simulink model "simQuadrotor"  (R2014b)
settings: Solver=ode45  StartTime=0.0  StopTime=tof  FixedStep=dt  MaxStep=dtmax  RelTol=1e-3
values from neighbouring files (symbols this model uses):
  a = (IzzT - IxxT)./ IxxT    [quadrotor.m]
  alpha = 1    [quadrotor.m]
  Aq = -20    [quadrotor.m]
  Ar = -10*eye(2)    [quadrotor.m]
  Arm = [-20 0 ; 0 -5]    [quadrotor.m]
  As = -50*eye(3)    [quadrotor.m]
  attitudeControlFlag = 4    [quadrotor.m]
  Bq = 1    [quadrotor.m]
  Br = [1 0]    [quadrotor.m]
  Dhat0 = zeros(3,1)    [quadrotor.m]
  Dlimit = 2.5    [quadrotor.m]
  DSecondLimit = 2    [quadrotor.m]
  dtFc = 10e-3    (= 0.01)    [quadrotor.m]
  epsilon = 0.1    [quadrotor.m]
  epsilontheta = 0.1    [quadrotor.m]
  euler0 = [0 0 0]'*pi/180    [quadrotor.m]
  Eulerc_ftc = [0 0 0]'    [quadrotor.m]
  faultyPropellerVec = double(not(faultyPropellerVec))    [quadrotor.m]
  FDstart = 3    [quadrotor.m]
  flims = [0.2*0 3.8*2.5]    [quadrotor.m]
  ftc_f2 = 0.1*2    (= 0.2)    [quadrotor.m]
  g = 9.81    [quadrotor.m]
  GammaW = 10000    [quadrotor.m]
  IxxB = IxxT - 4*IxxP    (= 0.0027)    [quadrotor.m]
  IxxT = 2.7e-3    (= 0.0027)    [quadrotor.m]
  IyyB = IyyT - 4*IyyP    (= 0.0027)    [quadrotor.m]
  IyyT = IxxT    (= 0.0027)    [quadrotor.m]
  IzzB = IzzT - 4*IzzP    (= 0.00514)    [quadrotor.m]
  IzzP = 1.5e-5    (= 1.5e-05)    [quadrotor.m]
  IzzT = 5.2e-3    (= 0.0052)    [quadrotor.m]
  Kdxx = 0.7e-4/10    (= 7e-06)    [quadrotor.m]
  Kdzz = 1.4e-4    (= 0.00014)    [quadrotor.m]
  Kf = 6.41e-6    (= 6.41e-06)    [quadrotor.m]
  Kp = 2*0.75*diag([1 1 1])    [quadrotor.m]
  Kp4 = 0.05    [quadrotor.m]
  Ktau = 1.72e-2    (= 0.0172)    [quadrotor.m]
  Kv = 0*0.005*diag([1 1 1])    [quadrotor.m]
  Kv4 = 0.02    [quadrotor.m]
  l = 0.17    [quadrotor.m]
  m = 0.5    [quadrotor.m]
  nc_ftc = 1    [quadrotor.m]
  nCheby = 3    [quadrotor.m]
  pqr0 = [0 0 0]'*pi/180    [quadrotor.m]
  Ps = lyap(As',Q)    [quadrotor.m]
  q0 = [euler0 ; pqr0]    [quadrotor.m]
  qp0 = 0    [quadrotor.m]
  sigmaMot = 0.015    [quadrotor.m]
  tfault = 5    [quadrotor.m]
  Vb0 = [0 0 0]'    [quadrotor.m]
  W0 = 0    [quadrotor.m]
  Wbnd = 10    [quadrotor.m]
  Xe0 = [0 0 0]'    [quadrotor.m]
  xhat0 = [pqr0]    [quadrotor.m]
undefined symbols (not defined in the file or in its folder): Intmax, Intmin, magnitude, rmax, rmin
libraries: aerolibutil x38, simulink x11, vrlib x3, dspbuff3 x1
(part 1 of 3)
settings Model: Creator=alp.marangoz  LastModifiedBy=alpmarangoz
settings SolverCC: AutoInsertRateTranBlk=on
settings DataIOCC: SignalLoggingSaveFormat=ModelDataLogs
settings OptimizationCC: ExpressionDepthLimit=2147483647
settings DebuggingCC: UnderspecifiedInitializationDetection=Classic  MergeDetectMultiDrivingBlocksExec=none  InheritedTsInSrcMsg=none  CheckMatrixSingularityMsg=error  FcnCallInpInsideContextMsg=UseLocalSettings  StateNameClashWarn=warning
settings GRTTargetCC: CombineOutputUpdateFcns=off  GRTInterface=on

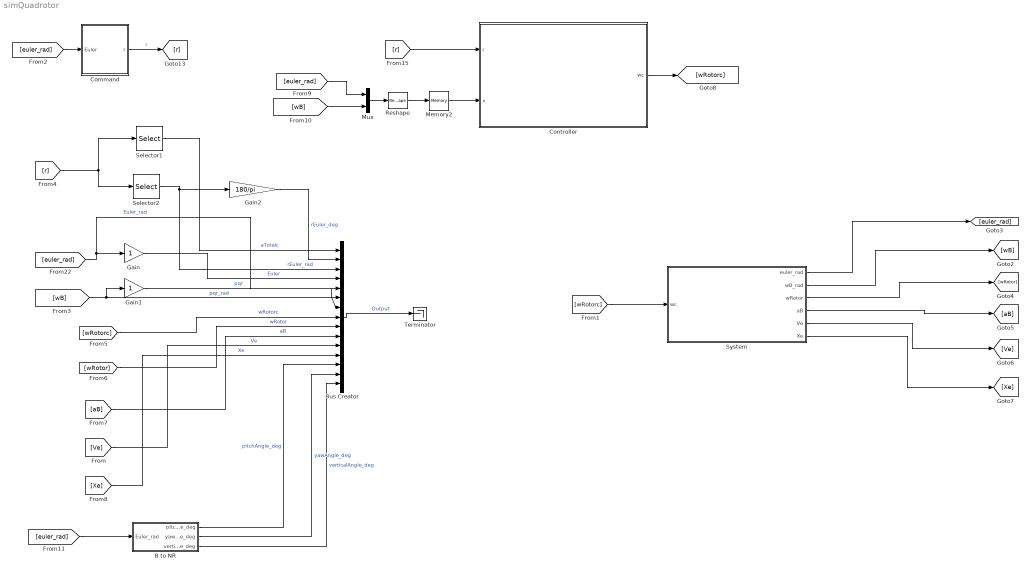
== system simQuadrotor ==
  B to NR : Subsystem  TreatAsAtomicUnit=on
  Bus Creator : BusCreator  Inputs=15
  Command : Subsystem  TreatAsAtomicUnit=on  SystemSampleTime=dtFc
  Controller : Subsystem  TreatAsAtomicUnit=on  SystemSampleTime=dtFc
  Gain : Gain
  Gain1 : Gain
  Gain2 : Gain  Gain=180/pi
  Memory2 : Memory  X0=q0  InheritSampleTime=on  LinearizeMemory=on  LinearizeAsDelay=on
  Mux : Mux  Inputs=2
  Reshape : Reshape  OutputDimensionality=Column vector (2-D)
  Selector1 : Selector  NumberOfDimensions=2  InputPortWidth=2  IndexOptions=Index vector (dialog),Index vector (dialog)  Indices=1,1  OutputSizes=1,1
  Selector2 : Selector  NumberOfDimensions=2  InputPortWidth=3  IndexOptions=Index vector (dialog),Index vector (dialog)  Indices=[2 3 4],1  OutputSizes=1,1
  System : Subsystem  TreatAsAtomicUnit=on
  Terminator : Terminator
  wires:
  Command/1(r) -> [r]  "r"
  Controller/1(wc) -> [wRotorc]
  [wRotorc] -> System/1(wc)
  Reshape/1 -> Memory2/1
  [euler_rad] -> Command/1(Euler)
  Memory2/1 -> Controller/2(x)
  [r] -> Controller/1(r)
  Bus Creator/1 -> Terminator/1  "Output"
  [r] -> Selector1/1, Selector2/1
  System/3(wRotor) -> [wRotor]
  System/4(aB) -> [aB]
  System/5(Ve) -> [Ve]
  System/6(Xe) -> [Xe]
  Selector1/1 -> Bus Creator/1  "aTotalc"
  Selector2/1 -> Gain2/1, Bus Creator/3  "rEuler_rad"
  [euler_rad] -> Gain/1, Bus Creator/5  "Euler_rad"
  [wRotorc] -> Bus Creator/8  "wRotorc"
  [wRotor] -> Bus Creator/9  "wRotor"
  [aB] -> Bus Creator/10  "aB"
  [Ve] -> Bus Creator/11  "Ve"
  [Xe] -> Bus Creator/12  "Xe"
  System/1(euler_rad) -> [euler_rad]
  System/2(wB_rad) -> [wB]
  Mux/1 -> Reshape/1
  [euler_rad] -> Mux/1
  [wB] -> Mux/2
  Gain/1 -> Bus Creator/4  "Euler"
  [wB] -> Bus Creator/7, Gain1/1  "pqr_rad"
  Gain1/1 -> Bus Creator/6  "pqr"
  [euler_rad] -> B to NR/1(Euler_rad)
  B to NR/1(pitchAngle_deg) -> Bus Creator/13  "pitchAngle_deg"
  B to NR/2(yawAngle_deg) -> Bus Creator/14  "yawAngle_deg"
  B to NR/3(verticalAngle_deg) -> Bus Creator/15  "verticalAngle_deg"
  Gain2/1 -> Bus Creator/2  "rEuler_deg"

== system simQuadrotor/B to NR ==
  Euler_rad : Inport
  Add : Sum
  Add1 : Sum  Inputs=+-
  Constant1 : Constant  Value=90  VectorParams1D=off
  Constant2 : Constant  Value=[0 0 1]'  VectorParams1D=off
  DCM E to B1 : Subsystem
  Gain : Gain  Gain=180/pi
  Gain1 : Gain  Gain=180/pi
  Math Function : Math  Operator=square  SaturateOnIntegerOverflow=on
  Math Function1 : Math  Operator=square  SaturateOnIntegerOverflow=on
  Math Function2 : Math  Operator=transpose  SaturateOnIntegerOverflow=on
  Product4 : Product  Multiplication=Matrix(*)  RndMeth=Zero
  Selector1 : Selector  InputPortWidth=3  Indices=3
  Selector2 : Selector  InputPortWidth=3  Indices=2
  Selector3 : Selector  InputPortWidth=3
  Sqrt : Sqrt  SaturateOnIntegerOverflow=on
  Trigonometric Function : Trigonometry  Operator=atan2
  Trigonometric Function1 : Trigonometry  Operator=atan2
  pitchAngle_deg : Outport
  yawAngle_deg : Outport  Port=2
  verticalAngle_deg : Outport  Port=3
  wires:
  Euler_rad/1 -> [phithetapsi]  "Euler_rad"
  Math Function2/1 -> [R]
  [phithetapsi] -> DCM E to B1/1(phithetapsi)
  DCM E to B1/1(CB_E) -> Math Function2/1
  [R] -> Product4/1
  Constant2/1 -> Product4/2
  Product4/1 -> [Gamma]
  [Gamma] -> Selector1/1, Selector3/1, Selector2/1
  Selector3/1 -> [u1]
  Selector2/1 -> [u2]
  Selector1/1 -> [u3]
  [u1] -> Math Function/1
  [u2] -> Math Function1/1
  Math Function/1 -> Add/1
  Math Function1/1 -> Add/2
  Add/1 -> Sqrt/1
  [u3] -> Trigonometric Function/1
  Sqrt/1 -> Trigonometric Function/2
  Trigonometric Function/1 -> Gain/1
  Trigonometric Function1/1 -> Gain1/1
  [u2] -> Trigonometric Function1/1
  [u1] -> Trigonometric Function1/2
  [yawAngle_deg] -> yawAngle_deg/1
  [pitchAngle_deg] -> pitchAngle_deg/1
  Gain/1 -> [pitchAngle_deg]
  Gain1/1 -> [yawAngle_deg]
  Constant1/1 -> Add1/2
  [pitchAngle_deg] -> Add1/1
  Add1/1 -> [verticalAngle_deg]
  [verticalAngle_deg] -> verticalAngle_deg/1

== system simQuadrotor/Command ==
  Euler : Inport
  From Workspace : FromWorkspace  VariableName=r  Interpolate=off  OutputAfterFinalValue=Setting to zero
  Memory2 : Memory  X0=euler0  InheritSampleTime=on  LinearizeMemory=on  LinearizeAsDelay=on
  Reshape1 : Reshape  OutputDimensionality=Column vector (2-D)
  Selector : Selector  NumberOfDimensions=2  InputPortWidth=2  IndexOptions=Index vector (dialog),Index vector (dialog)  Indices=1,1  OutputSizes=1,1
  Selector1 : Selector  NumberOfDimensions=2  InputPortWidth=3  IndexOptions=Index vector (dialog),Index vector (dialog)  Indices=[2 3 4],1  OutputSizes=1,1
  Subtract : Sum  Inputs=+-
  Terminator : Terminator
  Terminator1 : Terminator
  Terminator2 : Terminator
  r : Outport  InitialOutput=0
  wires:
  From Workspace/1 -> Reshape1/1
  Reshape1/1 -> r/1, Selector/1, Selector1/1
  Euler/1 -> Memory2/1
  Memory2/1 -> [euler]
  [euler] -> Subtract/2  "q"
  Selector/1 -> Terminator/1  "rnc"
  Selector1/1 -> Terminator2/1, Subtract/1  "rEuler"
  Subtract/1 -> Terminator1/1  "eEuler"

== system simQuadrotor/Controller ==
  r : Inport
  x : Inport  Port=2
  1 : Selector  NumberOfDimensions=2  InputPortWidth=4  IndexOptions=Index vector (dialog),Index vector (dialog)  Indices=[1],1  OutputSizes=1,1
  2 : Selector  NumberOfDimensions=2  InputPortWidth=4  IndexOptions=Index vector (dialog),Index vector (dialog)  Indices=[2 3 4],1  OutputSizes=1,1
  Disturbance Estimator : Subsystem
  FTC Controller : Subsystem  TreatAsAtomicUnit=on
  Fault Detection : Subsystem  TreatAsAtomicUnit=on
  Gain : Gain  Gain=180/pi
  Gain1 : Gain
  Logical Operator : Logic  Operator=NOT  AllPortsSameDT=off  OutDataTypeStr=boolean
  Memory1 : Memory  InheritSampleTime=on  LinearizeMemory=on  LinearizeAsDelay=on
  Memory2 : Memory  InheritSampleTime=on  LinearizeMemory=on  LinearizeAsDelay=on
  Memory3 : Memory  InheritSampleTime=on  LinearizeMemory=on  LinearizeAsDelay=on
  Nominal Controller : Subsystem  TreatAsAtomicUnit=on
  Reshape3 : Reshape  OutputDimensionality=Column vector (2-D)
  Switch : Switch  Criteria=u2 > Threshold
  Terminator : Terminator
  Terminator1 : Terminator
  Terminator2 : Terminator
  "[4 5 6]" : Selector  NumberOfDimensions=2  InputPortWidth=3  IndexOptions=Index vector (dialog),Index vector (dialog)  Indices=[4 5 6],1  OutputSizes=1,1
  wc : Outport
  wires:
  r/1 -> [r]  "r"
  x/1 -> [x]  "x"
  [wc] -> wc/1  "wc"
  [x] -> "[4 5 6]"/1
  "[4 5 6]"/1 -> Reshape3/1
  Reshape3/1 -> Terminator2/1  "pqr"
  Switch/1 -> [wc]
  [wcNominal] -> Switch/3
  [wcFTC] -> Gain1/1
  [faultDetected] -> Switch/2  "faultDetected"
  [r] -> 1/1, 2/1
  1/1 -> Terminator1/1  "nc"
  2/1 -> Gain/1
  Gain/1 -> Terminator/1  "Eulerc"
  [r] -> Nominal Controller/1(r)
  [x] -> Nominal Controller/2(x)
  Nominal Controller/1(wcNominal) -> [wcNominal]  "wcNominal"
  Logical Operator/1 -> Memory2/1
  Memory1/1 -> [enableFTC]
  Memory2/1 -> [enableNominal]
  [faultDetected] -> Logical Operator/1, Memory1/1
  [enableNominal] -> Nominal Controller/Enable
  [enableFTC] -> FTC Controller/Enable
  [x] -> FTC Controller/2(x)
  FTC Controller/1(wcFTC) -> [wcFTC]  "wcFTC"
  Gain1/1 -> Switch/1
  Disturbance Estimator/1(Dhat) -> [Dhat]
  [Dhat] -> Fault Detection/1(Dhat)
  Fault Detection/2(faultDetected) -> [faultDetected]
  [enableNominal] -> Disturbance Estimator/Enable
  Fault Detection/1(faultyRotor) -> [faultyRotor]
  [faultyRotor] -> FTC Controller/1(faultyRotor)
  [wc] -> Memory3/1
  Memory3/1 -> Disturbance Estimator/2(wc)
  [x] -> Disturbance Estimator/1(x)

== system simQuadrotor/System ==
  wc : Inport
  Demux : Demux
  Fault Insertion : Subsystem
  Flight Mechanics : Subsystem
  Gain7 : Gain  Gain=Kf
  Math Function7 : Math  Operator=magnitude^2  SaturateOnIntegerOverflow=on
  Motor Dynamics : Subsystem
  Navigation : Subsystem
  Reshape5 : Reshape  OutputDimensionality=Column vector (2-D)
  Terminator : Terminator
  euler_rad : Outport
  wB_rad : Outport  Port=2
  wRotor : Outport  Port=3
  aB : Outport  Port=4
  Ve : Outport  Port=5
  Xe : Outport  Port=6
  wires:
  wc/1 -> Reshape5/1
  Reshape5/1 -> [wc]  "wc"
  [euler_rad] -> euler_rad/1
  Flight Mechanics/1(aB) -> [aB], Navigation/1(axyz)
  Flight Mechanics/2(wB_rad) -> Navigation/2(wxyz), [wB]
  [wc] -> Demux/1
  Demux/1 -> Motor Dynamics/1(w1c)
  Demux/2 -> Motor Dynamics/2(w2c)
  Demux/3 -> Motor Dynamics/3(w3c)
  Demux/4 -> Motor Dynamics/4(w4c)
  [euler_rad] -> Flight Mechanics/5(Euler)
  Navigation/1(Ve) -> [Ve]
  Navigation/2(Xe) -> [Xe]
  Navigation/3(euler_rad) -> [euler_rad]
  [wRotor] -> wRotor/1
  [Xe] -> Xe/1
  [Ve] -> Ve/1
  [aB] -> aB/1
  Motor Dynamics/1(wRotor) -> Fault Insertion/1(wRotor)
  Fault Insertion/1(wRotor_app) -> Math Function7/1, [wRotor]
  Fault Insertion/5(w4) -> Flight Mechanics/4(w4)
  Fault Insertion/4(w3) -> Flight Mechanics/3(w3)
  Fault Insertion/3(w2) -> Flight Mechanics/2(w2)
  Fault Insertion/2(w1) -> Flight Mechanics/1(w1)
  [wB] -> wB_rad/1
  Gain7/1 -> Terminator/1  "frotorApp"
  Math Function7/1 -> Gain7/1

== system simQuadrotor/B to NR/DCM E to B1 ==
  phithetapsi : Inport
  Create 3x3 Matrix : aerolibutil/Create 3x3 Matrix
  Fcn11 : Fcn  Expr=u(5)*u(6)
  Fcn12 : Fcn  Expr=u(3)*u(5)
  Fcn13 : Fcn  Expr=-u(2)
  Fcn21 : Fcn  Expr=u(1)*u(2)*u(6)-u(4)*u(3)
  Fcn22 : Fcn  Expr=u(1)*u(2)*u(3)+u(4)*u(6)
  Fcn23 : Fcn  Expr=u(1)*u(5)
  Fcn31 : Fcn  Expr=u(4)*u(2)*u(6)+u(1)*u(3)
  Fcn32 : Fcn  Expr=u(4)*u(2)*u(3)-u(1)*u(6)
  Fcn33 : Fcn  Expr=u(4)*u(5)
  Mux : Mux  Inputs=2
  sincos : Trigonometry  Operator=sincos
  CB_E : Outport
  wires:
  Create 3x3 Matrix/1 -> CB_E/1  "CB_E"
  phithetapsi/1 -> sincos/1  "phithetapsi"
  Fcn33/1 -> Create 3x3 Matrix/9
  Fcn32/1 -> Create 3x3 Matrix/8
  Fcn23/1 -> Create 3x3 Matrix/6
  Fcn22/1 -> Create 3x3 Matrix/5
  Fcn31/1 -> Create 3x3 Matrix/7
  Fcn21/1 -> Create 3x3 Matrix/4
  Fcn13/1 -> Create 3x3 Matrix/3
  Fcn12/1 -> Create 3x3 Matrix/2
  Fcn11/1 -> Create 3x3 Matrix/1
  Mux/1 -> Fcn21/1, Fcn13/1, Fcn12/1, Fcn11/1, Fcn22/1, Fcn23/1, Fcn31/1, Fcn33/1, Fcn32/1
  sincos/2 -> Mux/2
  sincos/1 -> Mux/1

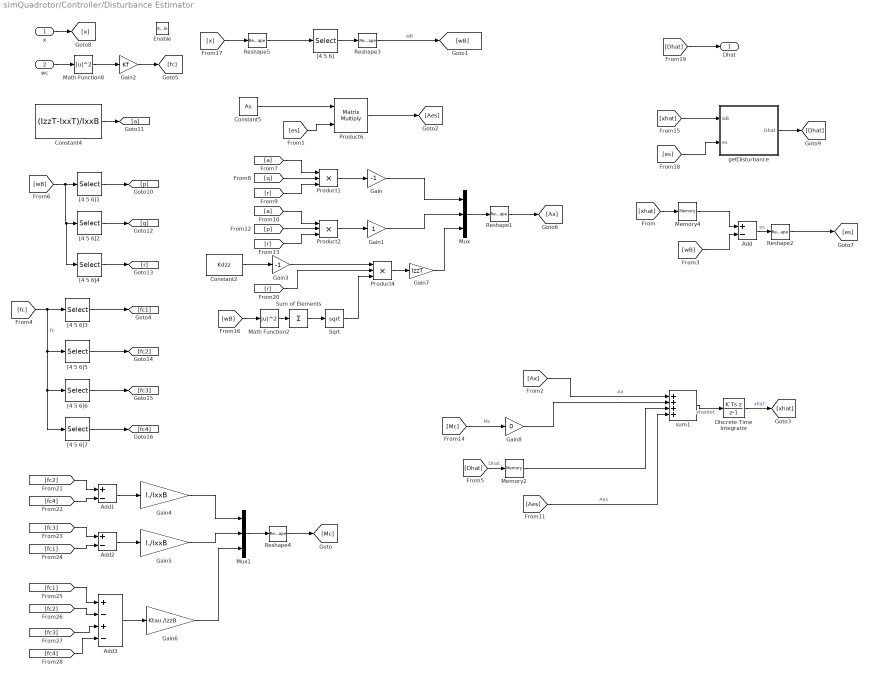
== system simQuadrotor/Controller/Disturbance Estimator ==
  x : Inport
  wc : Inport  Port=2
  Enable : EnablePort
  Add : Sum  Inputs=+-
  Add1 : Sum  Inputs=+-
  Add2 : Sum  Inputs=+-
  Add3 : Sum  Inputs=+-+-
  Constant2 : Constant  Value=Kdzz  VectorParams1D=off
  Constant4 : Constant  Value=(IzzT-IxxT)/IxxB  VectorParams1D=off
  Constant5 : Constant  Value=As
  Discrete-Time Integrator : DiscreteIntegrator  IntegratorMethod=Integration: Backward Euler  InitialCondition=xhat0  InitialConditionSetting=State (most efficient)  SampleTime=-1  UpperSaturationLimit=Intmax  LowerSaturationLimit=Intmin
  Gain : Gain  Gain=-1
  Gain1 : Gain
  Gain2 : Gain  Gain=Kf
  Gain3 : Gain  Gain=-1
  Gain4 : Gain  Gain=l./IxxB
  Gain5 : Gain  Gain=l./IxxB
  Gain6 : Gain  Gain=Ktau./IzzB
  Gain7 : Gain  Gain=IzzT
  Gain8 : Gain  Gain=0
  Math Function2 : Math  Operator=magnitude^2  SaturateOnIntegerOverflow=on
  Math Function8 : Math  Operator=magnitude^2  SaturateOnIntegerOverflow=on
  Memory2 : Memory  X0=Dhat0  InheritSampleTime=on  LinearizeMemory=on  LinearizeAsDelay=on
  Memory4 : Memory  X0=xhat0  InheritSampleTime=on  LinearizeMemory=on  LinearizeAsDelay=on
  Mux : Mux  Inputs=3
  Mux1 : Mux  Inputs=3
  Product1 : Product  Inputs=3  RndMeth=Zero
  Product2 : Product  Inputs=3  RndMeth=Zero
  Product4 : Product  Inputs=3  RndMeth=Zero
  Product6 : Product  Multiplication=Matrix(*)  RndMeth=Zero
  Reshape{1..5} (5 alike) : Reshape  OutputDimensionality=Column vector (2-D)
  Sqrt : Sqrt  SaturateOnIntegerOverflow=on
  Sum of Elements : Sum  Inputs=+
  "[4 5 6]" : Selector  NumberOfDimensions=2  InputPortWidth=3  IndexOptions=Index vector (dialog),Index vector (dialog)  Indices=[4 5 6],1  OutputSizes=1,1
  "[4 5 6]1" : Selector  InputPortWidth=3
  "[4 5 6]2" : Selector  InputPortWidth=3  Indices=2
  "[4 5 6]3" : Selector  InputPortWidth=4
  "[4 5 6]4" : Selector  InputPortWidth=3  Indices=3
  "[4 5 6]5" : Selector  InputPortWidth=4  Indices=2
  "[4 5 6]6" : Selector  InputPortWidth=4  Indices=3
  "[4 5 6]7" : Selector  InputPortWidth=4  Indices=4
  getDisturbance : Subsystem
  sum1 : Sum  Inputs=++++
  Dhat : Outport
  wires:
  [xhat] -> getDisturbance/1(wB)
  [es] -> getDisturbance/2(es)
  getDisturbance/1(Dhat) -> [Dhat]
  [Dhat] -> Dhat/1
  Constant4/1 -> [a]
  x/1 -> [x]
  [x] -> Reshape5/1
  "[4 5 6]"/1 -> Reshape3/1
  Reshape5/1 -> "[4 5 6]"/1
  Reshape3/1 -> [wB]  "wB"
  Product6/1 -> [Aes]
  Constant5/1 -> Product6/1
  [es] -> Product6/2
  Reshape2/1 -> [es]
  [xhat] -> Memory4/1
  [wB] -> Add/2
  Add/1 -> Reshape2/1  "es"
  Memory4/1 -> Add/1
  [Dhat] -> Memory2/1  "Dhat"
  [Ax] -> sum1/1  "Ax"
  sum1/1 -> Discrete-Time Integrator/1  "xhatdot"
  Discrete-Time Integrator/1 -> [xhat]  "xhat"
  [wB] -> "[4 5 6]4"/1, "[4 5 6]2"/1, "[4 5 6]1"/1
  "[4 5 6]2"/1 -> [q]
  "[4 5 6]1"/1 -> [p]
  "[4 5 6]4"/1 -> [r]
  Reshape1/1 -> [Ax]
  Mux/1 -> Reshape1/1
  [q] -> Product1/2
  [r] -> Product1/3
  [a] -> Product1/1
  [p] -> Product2/2
  [r] -> Product2/3
  [a] -> Product2/1
  Product1/1 -> Gain/1
  Gain/1 -> Mux/1
  Product2/1 -> Gain1/1
  Gain1/1 -> Mux/2
  Product4/1 -> Gain7/1
  [Mc] -> Gain8/1  "Mc"
  wc/1 -> Math Function8/1
  Math Function8/1 -> Gain2/1
  Gain2/1 -> [fc]
  Memory2/1 -> sum1/3
  [Aes] -> sum1/4  "Aes"
  [r] -> Product4/2
  Gain3/1 -> Product4/1
  Constant2/1 -> Gain3/1
  Math Function2/1 -> Sum of Elements/1
  Sum of Elements/1 -> Sqrt/1
  [wB] -> Math Function2/1
  Sqrt/1 -> Product4/3
  Reshape4/1 -> [Mc]
  Mux1/1 -> Reshape4/1
  [fc] -> "[4 5 6]7"/1, "[4 5 6]6"/1, "[4 5 6]5"/1, "[4 5 6]3"/1  "fc"
  "[4 5 6]3"/1 -> [fc1]
  "[4 5 6]5"/1 -> [fc2]
  "[4 5 6]6"/1 -> [fc3]
  "[4 5 6]7"/1 -> [fc4]
  [fc2] -> Add1/1
  [fc4] -> Add1/2
  Add1/1 -> Gain4/1
  Gain4/1 -> Mux1/1
  [fc3] -> Add2/1
  [fc1] -> Add2/2
  Add2/1 -> Gain5/1
  Gain5/1 -> Mux1/2
  [fc1] -> Add3/1
  [fc2] -> Add3/2
  Add3/1 -> Gain6/1
  [fc3] -> Add3/3
  [fc4] -> Add3/4
  Gain6/1 -> Mux1/3
  Gain7/1 -> Mux/3
  Gain8/1 -> sum1/2

== system simQuadrotor/Controller/FTC Controller ==
  faultyRotor : Inport
  x : Inport  Port=2
  Enable : EnablePort
  Compare To Constant : simulink/Logic and Bit Operations/Compare To Constant  relop===  const=1  OutDataTypeStr=boolean
  Constant : Constant  Value=Eulerc_ftc  VectorParams1D=off
  Constant1 : Constant  Value=nc_ftc  VectorParams1D=off
  Ground : Ground
  Multiport Switch : MultiPortSwitch  Inputs=2
  Mux : Mux  Inputs=2
  Propeller Rotation Rate Calculation : Subsystem
  Reshape : Reshape  OutputDimensionality=Column vector (2-D)
  SingleProp Compensation : Subsystem  TreatAsAtomicUnit=on  SystemSampleTime=dtFc
  Sum of Elements : Sum  Inputs=+
  Sum of Elements2 : Sum  Inputs=+
  wcFTC : Outport
  wires:
  x/1 -> [x]
  Propeller Rotation Rate Calculation/1(wc) -> [wcFTC]
  [wcFTC] -> wcFTC/1
  Sum of Elements/1 -> Compare To Constant/1
  SingleProp Compensation/1(fic) -> [ficSp]
  [faultyRotor] -> Sum of Elements/1
  Compare To Constant/1 -> SingleProp Compensation/Enable  "spEnable"
  [faultyRotor] -> Sum of Elements2/1
  Sum of Elements2/1 -> Multiport Switch/1  "FaultCase"
  [ficSp] -> Multiport Switch/2  "ficSp"
  Multiport Switch/1 -> Propeller Rotation Rate Calculation/1(fic)
  Ground/1 -> Multiport Switch/3  "ficDp"
  faultyRotor/1 -> [faultyRotor]  "faultyRotor"
  Constant1/1 -> Mux/1
  Constant/1 -> Mux/2
  Mux/1 -> Reshape/1
  Reshape/1 -> [rFTC]  "rFTC"
  [rFTC] -> SingleProp Compensation/1(r)
  [x] -> SingleProp Compensation/2(x)
  [faultyRotor] -> SingleProp Compensation/3(faultyRotor)

== system simQuadrotor/Controller/Fault Detection ==
  Dhat : Inport
  Abs : Abs
  Compare To Constant : simulink/Logic and Bit Operations/Compare To Constant  relop=>=  const=Dlimit  OutDataTypeStr=boolean
  Compare To Constant1 : simulink/Logic and Bit Operations/Compare To Constant  relop=>=  const=FDstart  OutDataTypeStr=boolean
  Compare To Constant2 : simulink/Logic and Bit Operations/Compare To Constant  relop=>=  const=DSecondLimit  OutDataTypeStr=uint8
  Digital Clock : DigitalClock  SampleTime=-1
  Find Rotor : Subsystem  TreatAsAtomicUnit=on
  Logical Operator : Logic  AllPortsSameDT=off  OutDataTypeStr=boolean
  Product : Product
  Product1 : Product
  Sign : Signum
  Sum of Elements : Sum  Inputs=+
  Triggered step : Subsystem
  faultyRotor : Outport
  faultDetected : Outport  Port=2
  wires:
  Abs/1 -> Compare To Constant2/1, Compare To Constant/1
  Dhat/1 -> Sign/1, Abs/1
  Compare To Constant/1 -> Sum of Elements/1
  Sum of Elements/1 -> Logical Operator/1
  Logical Operator/1 -> Triggered step/Trigger
  Digital Clock/1 -> Compare To Constant1/1
  Compare To Constant1/1 -> Logical Operator/2
  [faultDetected] -> faultDetected/1  "faultDetected"
  Triggered step/1(Out1) -> [faultDetected]
  Sign/1 -> Product/1
  Compare To Constant2/1 -> Product/2
  Product/1 -> [Dsigns]  "DSigns"
  [faultDetected] -> Product1/1
  [Dsigns] -> Find Rotor/1(Dsigns)
  Product1/1 -> faultyRotor/1  "faultyRotor"
  Find Rotor/1(faultyRotor) -> Product1/2

== system simQuadrotor/Controller/Nominal Controller ==
  r : Inport
  x : Inport  Port=2
  Enable : EnablePort
  1 : Selector  NumberOfDimensions=2  InputPortWidth=4  IndexOptions=Index vector (dialog),Index vector (dialog)  Indices=[1],1  OutputSizes=1,1
  Constant : Constant  Value=attitudeControlFlag  VectorParams1D=off
  Gain1 : Gain
  Index Vector : MultiPortSwitch  DataPortOrder=Zero-based contiguous  Inputs=5  zeroidx=on
  Motor Force Calculation : Subsystem  TreatAsAtomicUnit=on
  PD-Attitude Control with wB_IB : Subsystem  TreatAsAtomicUnit=on
  PD-control for Attitude : Subsystem  TreatAsAtomicUnit=on
  PD-control for AttitudeAlt : Subsystem  TreatAsAtomicUnit=on
  PD-control for Reduced Attitude : Subsystem  TreatAsAtomicUnit=on
  PD-control for Reduced Attitude-Bullo : Subsystem  TreatAsAtomicUnit=on
  Propeller Rotation Rate Calculation : Subsystem
  Required Total Thrust : Subsystem  TreatAsAtomicUnit=on
  wcNominal : Outport
  wires:
  [wcNominal] -> wcNominal/1
  [Mc] -> Motor Force Calculation/2(Mc)  "Mc"
  Propeller Rotation Rate Calculation/1(wc) -> [wcNominal]
  [fc] -> Motor Force Calculation/1(fc)  "fc"
  Motor Force Calculation/1(fic) -> Propeller Rotation Rate Calculation/1(fic)  "fic"
  [x] -> PD-control for Attitude/2(q)
  [r] -> PD-control for Attitude/1(r)
  [r] -> 1/1
  Gain1/1 -> Required Total Thrust/1(q)
  1/1 -> Required Total Thrust/2(nc)
  Required Total Thrust/1(fc) -> [fc]
  [x] -> Gain1/1
  x/1 -> [x]
  r/1 -> [r]  "r"
  Constant/1 -> Index Vector/1
  PD-control for Reduced Attitude/1(Mc) -> Index Vector/2  "McReducedAttitude"
  PD-control for Attitude/1(Mc) -> Index Vector/3  "McFullAttitude"
  Index Vector/1 -> [Mc]
  [x] -> PD-control for Reduced Attitude/2(q)
  [r] -> PD-control for Reduced Attitude/1(r)
  [x] -> PD-Attitude Control with wB_IB/2(q)
  [r] -> PD-Attitude Control with wB_IB/1(r)
  [x] -> PD-control for AttitudeAlt/2(q)
  [r] -> PD-control for AttitudeAlt/1(r)
  PD-control for AttitudeAlt/1(Mc) -> Index Vector/4  "Mc_Omega_R_"
  PD-Attitude Control with wB_IB/1(Mc) -> Index Vector/5  "Mc_with_wB_IB"
  PD-control for Reduced Attitude-Bullo/1(Mc) -> Index Vector/6  "Mc_red_bullo"
  [r] -> PD-control for Reduced Attitude-Bullo/1(r)
  [x] -> PD-control for Reduced Attitude-Bullo/2(x)

== system simQuadrotor/System/Fault Insertion ==
  wRotor : Inport
  Clock : Clock
  Constant1 : Constant  Value=faultyPropellerVec  VectorParams1D=off
  Constant4 : Constant  Value=tfault
  Demux : Demux
  Ground2 : Ground
  MinMax1 : MinMax  Function=max  Inputs=2
  Product : Product
  Reshape : Reshape  OutputDimensionality=Column vector (2-D)
  Reshape1 : Reshape  OutputDimensionality=Column vector (2-D)
  Sign : Signum
  Subtract1 : Sum  Inputs=+-
  Switch2 : Switch  Criteria=u2 > Threshold
  wRotor_app : Outport
  w1 : Outport  Port=2
  w2 : Outport  Port=3
  w3 : Outport  Port=4
  w4 : Outport  Port=5
  wires:
  Clock/1 -> [time]
  MinMax1/1 -> [faultInsertion]  "faultInsertion"
  Sign/1 -> MinMax1/1
  Ground2/1 -> MinMax1/2
  Subtract1/1 -> Sign/1
  Constant4/1 -> Subtract1/2
  [time] -> Subtract1/1
  wRotor/1 -> [wRotor]  "wRotor"
  [faultInsertion] -> Switch2/2
  [wRotor_faulty] -> Switch2/1
  [wRotor] -> Switch2/3
  Switch2/1 -> Demux/1, wRotor_app/1  "wRotor_app"
  Product/1 -> [wRotor_faulty]
  [wRotor] -> Reshape1/1
  [w1] -> w1/1  "w1"
  [w2] -> w2/1  "w2"
  [w3] -> w3/1  "w3"
  [w4] -> w4/1  "w4"
  Demux/1 -> [w1]
  Demux/2 -> [w2]
  Demux/3 -> [w3]
  Demux/4 -> [w4]
  Reshape/1 -> Product/1
  Constant1/1 -> Reshape/1
  Reshape1/1 -> Product/2

== system simQuadrotor/System/Flight Mechanics ==
  w1 : Inport
  w2 : Inport  Port=2
  w3 : Inport  Port=3
  w4 : Inport  Port=4
  Euler : Inport  Port=5
  Attitude Dynamics : Subsystem
  DCM E to B : Subsystem
  Gain : Gain  Gain=180/pi
  Gain1 : Gain  Gain=1/g
  Mux : Mux  Inputs=3
  Mux1 : Mux  Inputs=3
  Reshape : Reshape  OutputDimensionality=Column vector (2-D)
  Reshape1 : Reshape  OutputDimensionality=Column vector (2-D)
  Terminator2 : Terminator
  Terminator7 : Terminator
  Translation Dynamics : Subsystem
  aB : Outport
  wB_rad : Outport  Port=2
  wires:
  Attitude Dynamics/1(p) -> Mux/1
  Attitude Dynamics/2(q) -> Mux/2
  Attitude Dynamics/3(r) -> Mux/3
  Translation Dynamics/1(ax) -> Mux1/1
  Translation Dynamics/2(ay) -> Mux1/2
  Translation Dynamics/3(az) -> Mux1/3
  Mux/1 -> Reshape/1
  Mux1/1 -> Reshape1/1
  Reshape1/1 -> [aB]
  Reshape/1 -> [wB]
  [w1] -> Attitude Dynamics/1(w1)
  [w2] -> Attitude Dynamics/2(w2)
  [w3] -> Attitude Dynamics/3(w3)
  [w4] -> Attitude Dynamics/4(w4)
  [w1] -> Translation Dynamics/1(w1)
  [w2] -> Translation Dynamics/2(w2)
  [w3] -> Translation Dynamics/3(w3)
  [w4] -> Translation Dynamics/4(w4)
  [wB] -> wB_rad/1, Gain/1  "wB_rad"
  [aB] -> aB/1, Gain1/1  "aB"
  w4/1 -> [w4]  "w4"
  w3/1 -> [w3]  "w3"
  w2/1 -> [w2]  "w2"
  w1/1 -> [w1]  "w1"
  [DCM_E_to_B] -> Translation Dynamics/5(DCM)
  [phithetapsi] -> DCM E to B/1(phithetapsi)
  Euler/1 -> [phithetapsi]
  Gain/1 -> Terminator7/1  "wB_deg"
  Gain1/1 -> Terminator2/1  "aB_g"
  DCM E to B/1(CB_E) -> [DCM_E_to_B]

== system simQuadrotor/System/Motor Dynamics ==
  w1c : Inport
  w2c : Inport  Port=2
  w3c : Inport  Port=3
  w4c : Inport  Port=4
  Gain{1,3,5,7} (4 alike) : Gain  Gain=Kf
  Gain{2,4,6,8} (4 alike) : Gain  Gain=1/Kf
  Math Function{1..2,4,6} (4 alike) : Math  Operator=sqrt  SaturateOnIntegerOverflow=on
  Math Function{3,5,7..8} (4 alike) : Math  Operator=magnitude^2  SaturateOnIntegerOverflow=on
  Mux : Mux
  Mux1 : Mux
  Mux2 : Mux
  Reshape2 : Reshape  OutputDimensionality=Column vector (2-D)
  Saturation{,1..3} (4 alike) : Saturate  UpperLimit=flims(2)  LowerLimit=flims(1)  ZeroCross=off
  Terminator : Terminator
  Terminator1 : Terminator
  Transfer Fcn{,1..3} (4 alike) : TransferFcn  Denominator=[sigmaMot 1]
  wRotor : Outport
  wires:
  w4c/1 -> [w4c], Mux1/4  "w4c"
  w3c/1 -> [w3c], Mux1/3  "w3c"
  w2c/1 -> [w2c], Mux1/2  "w2c"
  w1c/1 -> [w1c], Mux1/1  "w1c"
  [w1] -> Mux2/1  "w1"
  [w2] -> Mux2/2  "w2"
  [w3] -> Mux2/3  "w3"
  [w4] -> Mux2/4  "w4"
  [w1c] -> Transfer Fcn/1
  Transfer Fcn/1 -> Math Function8/1
  Math Function8/1 -> Gain1/1
  Gain1/1 -> Saturation/1  "f1d"
  Saturation/1 -> Gain2/1, Mux/1  "f1"
  Gain2/1 -> Math Function1/1
  Math Function1/1 -> [w1]
  [w2c] -> Transfer Fcn1/1
  Transfer Fcn1/1 -> Math Function3/1
  Math Function3/1 -> Gain3/1
  Gain3/1 -> Saturation1/1  "f2d"
  Saturation1/1 -> Gain4/1, Mux/2  "f2"
  Gain4/1 -> Math Function2/1
  Math Function2/1 -> [w2]
  [w3c] -> Transfer Fcn2/1
  Transfer Fcn2/1 -> Math Function5/1
  Math Function5/1 -> Gain5/1
  Gain5/1 -> Saturation2/1  "f3d"
  Saturation2/1 -> Gain6/1, Mux/3  "f3"
  Gain6/1 -> Math Function4/1
  Math Function4/1 -> [w3]
  [w4c] -> Transfer Fcn3/1
  Transfer Fcn3/1 -> Math Function7/1
  Math Function7/1 -> Gain7/1
  Gain7/1 -> Saturation3/1  "f4d"
  Saturation3/1 -> Gain8/1, Mux/4  "f4"
  Gain8/1 -> Math Function6/1
  Math Function6/1 -> [w4]
  Mux/1 -> Terminator/1  "frotor"
  Mux1/1 -> Terminator1/1  "wc"
  Reshape2/1 -> wRotor/1  "w"
  Mux2/1 -> Reshape2/1

== system simQuadrotor/System/Navigation ==
  axyz : Inport
  wxyz : Inport  Port=2
  3x3 Cross Product : aerolibutil/3x3 Cross Product
  Add : Sum  Inputs=+-
  Constant5 : Constant  Value=2*pi
  DCM E to B : Subsystem
  Fcn : Fcn  Expr=u[1]+(u[2]*u[4]+u[3]*u[7])*(u[5]/u[8])
  Fcn1 : Fcn  Expr=u[2]*u[7]-u[3]*u[4]
  Fcn2 : Fcn  Expr=(u[2]*u[4]+u[3]*u[7])/u[8]
  Integrator1 : Integrator  InitialCondition=euler0
  Integrator2 : Integrator  InitialCondition=Vb0
  Integrator3 : Integrator  InitialCondition=Xe0
  Math Function2 : Math  Operator=rem  SaturateOnIntegerOverflow=on
  Mux3 : Mux  Inputs=3
  Mux4 : Mux  Inputs=3
  Product1 : Product  Multiplication=Matrix(*)  RndMeth=Zero
  Product2 : Product  Inputs=/  Multiplication=Matrix(*)  RndMeth=Zero
  Trigonometric Function : Trigonometry  Operator=sincos
  Ve : Outport
  Xe : Outport  Port=2
  euler_rad : Outport  Port=3
  wires:
  axyz/1 -> [axyz]
  wxyz/1 -> [wxyz]
  [phithetapsi] -> euler_rad/1  "Euler"
  [Ve] -> Ve/1  "Ve"
  [Xe] -> Xe/1  "Xe"
  [wxyz] -> Mux3/1
  Trigonometric Function/1 -> Mux3/2
  Trigonometric Function/2 -> Mux3/3
  [phithetapsi] -> Trigonometric Function/1
  Mux3/1 -> Fcn1/1, Fcn/1, Fcn2/1
  Fcn/1 -> Mux4/1
  Fcn1/1 -> Mux4/2
  Fcn2/1 -> Mux4/3
  Mux4/1 -> Integrator1/1
  Integrator1/1 -> Math Function2/1
  Constant5/1 -> Math Function2/2
  Math Function2/1 -> [phithetapsi]
  [wxyz] -> 3x3 Cross Product/1
  [Vb] -> 3x3 Cross Product/2
  [axyz] -> Add/1
  3x3 Cross Product/1 -> Add/2
  Add/1 -> Integrator2/1
  Integrator2/1 -> [Vb], Product1/2
  [DCM_b_2_e] -> Product1/1
  Product1/1 -> [Ve], Integrator3/1
  Integrator3/1 -> [Xe]
  [phithetapsi] -> DCM E to B/1(phithetapsi)
  DCM E to B/1(CB_E) -> Product2/1
  Product2/1 -> [DCM_b_2_e]

== system simQuadrotor/Controller/Disturbance Estimator/getDisturbance ==
  wB : Inport
  es : Inport  Port=2
  Chebyshev Basis Functions : Subsystem
  getDhat : Subsystem  TreatAsAtomicUnit=on
  Dhat : Outport
  wires:
  [Dhat] -> Dhat/1  "Dhat"
  wB/1 -> [wB]
  es/1 -> [es]
  [basisSet] -> getDhat/1(psiz)  "basisSet"
  [es] -> getDhat/2(es)
  getDhat/1(Dhat) -> [Dhat]  "Dhat"
  Chebyshev Basis Functions/1(Tn) -> [Tnz]  "Tn"
  [wB] -> Chebyshev Basis Functions/1(x)
  [Tnz] -> [basisSet]

== system simQuadrotor/Controller/FTC Controller/Propeller Rotation Rate Calculation ==
  fic : Inport
  Constant3 : Constant  Value=Kf
  Divide : Product  Inputs=*/
  Math Function : Math  Operator=sqrt  SaturateOnIntegerOverflow=on
  wc : Outport
  wires:
  fic/1 -> [fic]
  [wc] -> wc/1
  [fic] -> Divide/1
  Constant3/1 -> Divide/2
  Divide/1 -> Math Function/1
  Math Function/1 -> [wc]

== system simQuadrotor/Controller/FTC Controller/SingleProp Compensation ==
  r : Inport
  x : Inport  Port=2
  faultyRotor : Inport  Port=3
  Enable : EnablePort
  1 : Selector  NumberOfDimensions=2  InputPortWidth=4  IndexOptions=Index vector (dialog),Index vector (dialog)  Indices=[1],1  OutputSizes=1,1
  Gain{1,3..6} (5 alike) : Gain
  Gain2 : Gain  Gain=1/IyyT
  Motor Force Calculation : Subsystem  TreatAsAtomicUnit=on
  PD-control for Reduced Attitude-Bullo : Subsystem  TreatAsAtomicUnit=on
  Perturbation Calculation : Subsystem  TreatAsAtomicUnit=on
  Required Total Thrust : Subsystem  TreatAsAtomicUnit=on
  Terminator : Terminator
  "[4 5 6]" : Selector  InputPortWidth=3  Indices=2
  w3 Controller : Subsystem  TreatAsAtomicUnit=on
  fic : Outport
  wires:
  Gain5/1 -> w3 Controller/2(qp)
  Gain4/1 -> w3 Controller/3(qc)
  Gain3/1 -> [u]
  Gain2/1 -> [qc]  "qc"
  "[4 5 6]"/1 -> Gain2/1
  [Mc] -> "[4 5 6]"/1
  [qc] -> Gain4/1
  [qp] -> Gain5/1
  PD-control for Reduced Attitude-Bullo/1(Mc) -> [Mc]  "Mc_ratt"
  [r] -> PD-control for Reduced Attitude-Bullo/1(r)
  [x] -> PD-control for Reduced Attitude-Bullo/2(x)
  [x] -> Perturbation Calculation/1(x)
  w3 Controller/1(Mc) -> Gain3/1  "u"
  [x] -> w3 Controller/1(x)
  [u] -> Motor Force Calculation/2(u)  "u"
  Perturbation Calculation/1(qp) -> [qp]  "qp"
  Required Total Thrust/1(fc) -> [fc]
  faultyRotor/1 -> Terminator/1
  1/1 -> Required Total Thrust/2(nc)  "nc"
  [r] -> 1/1
  Gain1/1 -> Required Total Thrust/1(x)
  [x] -> Gain1/1
  Motor Force Calculation/1(fic) -> fic/1
  [fc] -> Motor Force Calculation/1(fc)  "fc"
  x/1 -> [x]  "x"
  r/1 -> [r]  "r"
  [qc] -> Gain6/1
  Gain6/1 -> Perturbation Calculation/2(qc)

== system simQuadrotor/Controller/Fault Detection/Find Rotor ==
  Dsigns : Inport
  Compare To Zero : simulink/Logic and Bit Operations/Compare To Zero  relop===  OutDataTypeStr=boolean
  Compare To Zero1 : simulink/Logic and Bit Operations/Compare To Zero  relop=<  OutDataTypeStr=boolean
  Compare To Zero2 : simulink/Logic and Bit Operations/Compare To Zero  relop=<  OutDataTypeStr=boolean
  Compare To Zero3 : simulink/Logic and Bit Operations/Compare To Zero  relop=>  OutDataTypeStr=boolean
  Compare To Zero4 : simulink/Logic and Bit Operations/Compare To Zero  relop=>  OutDataTypeStr=boolean
  Compare To Zero5 : simulink/Logic and Bit Operations/Compare To Zero  relop=>  OutDataTypeStr=boolean
  Compare To Zero6 : simulink/Logic and Bit Operations/Compare To Zero  relop=<  OutDataTypeStr=boolean
  Constant1 : Constant  Value=faultyPropellerVec  VectorParams1D=off
  Data Type Conversion : DataTypeConversion  OutDataTypeStr=double
  Data Type Conversion1 : DataTypeConversion  OutDataTypeStr=double
  Demux : Demux  Outputs=3
  Logical Operator : Logic  Operator=NOT  AllPortsSameDT=off  OutDataTypeStr=boolean
  Mux : Mux
  Mux1 : Mux
  Reshape : Reshape  OutputDimensionality=Column vector (2-D)
  Reshape1 : Reshape  OutputDimensionality=Column vector (2-D)
  Switch : Switch  Criteria=u2 > Threshold
  Terminator : Terminator
  faultyRotor : Outport
  wires:
  Dsigns/1 -> Demux/1  "Dsigns"
  Demux/1 -> [D1]
  Demux/2 -> [D2]
  Demux/3 -> [D3]
  [D3] -> Compare To Zero/1
  [D1] -> Compare To Zero1/1
  [D2] -> Compare To Zero2/1
  [faultCase2] -> Switch/3
  [D1] -> Compare To Zero3/1
  [D2] -> Compare To Zero4/1
  Switch/1 -> Data Type Conversion/1
  Mux/1 -> [faultCase1]  "faultCase1"
  Compare To Zero2/1 -> Mux/3
  Compare To Zero3/1 -> Mux/4
  Compare To Zero1/1 -> Mux/2
  Compare To Zero4/1 -> Mux/1
  Mux1/1 -> [faultCase2]  "faultCase2"
  [D3] -> Compare To Zero5/1
  [D3] -> Compare To Zero6/1
  Compare To Zero5/1 -> Mux1/4, Mux1/2
  Compare To Zero6/1 -> Mux1/3, Mux1/1
  Data Type Conversion/1 -> Reshape/1
  Compare To Zero/1 -> Switch/2  "D3Sign"
  [faultCase1] -> Switch/1
  Constant1/1 -> Logical Operator/1
  Logical Operator/1 -> Data Type Conversion1/1
  Data Type Conversion1/1 -> Reshape1/1
  Reshape1/1 -> faultyRotor/1  "faultyRotor"
  Reshape/1 -> Terminator/1  "_faultyRotor"

== system simQuadrotor/Controller/Fault Detection/Triggered step ==
  Trigger : TriggerPort  PortDimensions=1
  Constant : Constant
  Out1 : Outport  InitialOutput=0
  wires:
  Constant/1 -> Out1/1

== system simQuadrotor/Controller/Nominal Controller/Motor Force Calculation ==
  fc : Inport
  Mc : Inport  Port=2
  Add : Sum  Inputs=+++
  Constant : Constant  Value=ones(4,1)
  Demux : Demux  Outputs=3
  Gain : Gain  Gain=1/4
  Gain{1,4,6,8} (4 alike) : Gain  Gain=-1/2
  Gain10 : Gain  Gain=1/Ktau
  Gain11 : Gain  Gain=1/l
  Gain{2..3,5,7} (4 alike) : Gain  Gain=1/2
  Gain9 : Gain  Gain=1/l
  Mux : Mux
  Mux1 : Mux
  Product : Product  Multiplication=Matrix(*)  RndMeth=Zero
  Reshape : Reshape  OutputDimensionality=Column vector (2-D)
  Reshape1 : Reshape  OutputDimensionality=Column vector (2-D)
  fic : Outport
  wires:
  Gain10/1 -> [df1234]
  Gain11/1 -> [df13]  "df13"
  Gain9/1 -> [df24]  "df24"
  Product/1 -> [fbar]
  Gain/1 -> Product/2
  Constant/1 -> Product/1
  Add/1 -> [fic]
  Demux/3 -> Gain10/1
  Demux/2 -> Gain11/1
  Demux/1 -> Gain9/1
  [Mc] -> Demux/1
  Reshape1/1 -> Add/3  "dfr"
  Mux1/1 -> Reshape1/1
  Gain8/1 -> Mux1/4
  Gain7/1 -> Mux1/3
  Gain6/1 -> Mux1/2
  Gain5/1 -> Mux1/1
  [df1234] -> Gain8/1
  [df1234] -> Gain7/1
  [df1234] -> Gain6/1
  [df1234] -> Gain5/1
  Gain4/1 -> Mux/4
  Gain3/1 -> Mux/3
  Gain2/1 -> Mux/2
  Gain1/1 -> Mux/1
  [df24] -> Gain4/1
  [df13] -> Gain3/1
  [df24] -> Gain2/1
  [df13] -> Gain1/1
  Mux/1 -> Reshape/1
  Reshape/1 -> Add/2  "dfpq"
  [fbar] -> Add/1  "fbar"
  [fc] -> Gain/1
  [fic] -> fic/1
  fc/1 -> [fc]
  Mc/1 -> [Mc]

== system simQuadrotor/Controller/Nominal Controller/PD-Attitude Control with wB_IB ==
  r : Inport
  q : Inport  Port=2
  Add3 : Sum
  Gain : Gain  Gain=Kv  Multiplication=Matrix(K*u)
  Gain2 : Gain  Gain=-1
  Gain4 : Gain  Gain=-Kp  Multiplication=Matrix(K*u)
  Reshape3 : Reshape  OutputDimensionality=Column vector (2-D)
  Reshape5 : Reshape  OutputDimensionality=Column vector (2-D)
  "[4 5 6]" : Selector  NumberOfDimensions=2  InputPortWidth=3  IndexOptions=Index vector (dialog),Index vector (dialog)  Indices=[4 5 6],1  OutputSizes=1,1
  get eR : Subsystem  TreatAsAtomicUnit=on
  Mc : Outport
  wires:
  q/1 -> [q]  "q"
  r/1 -> [r]  "r"
  [Mc] -> Mc/1
  Reshape3/1 -> [wB]  "wB"
  Gain/1 -> Gain2/1
  [wB] -> Gain/1
  Gain2/1 -> Add3/1  "D term"
  [wB_IBcommand] -> Add3/2  "E term"
  Reshape5/1 -> "[4 5 6]"/1
  "[4 5 6]"/1 -> Reshape3/1
  [q] -> Reshape5/1
  get eR/1(eR) -> [eR]
  [r] -> get eR/1(r)
  [q] -> get eR/2(q)
  [eR] -> Gain4/1
  Gain4/1 -> [wB_IBcommand]
  Add3/1 -> [Mc]

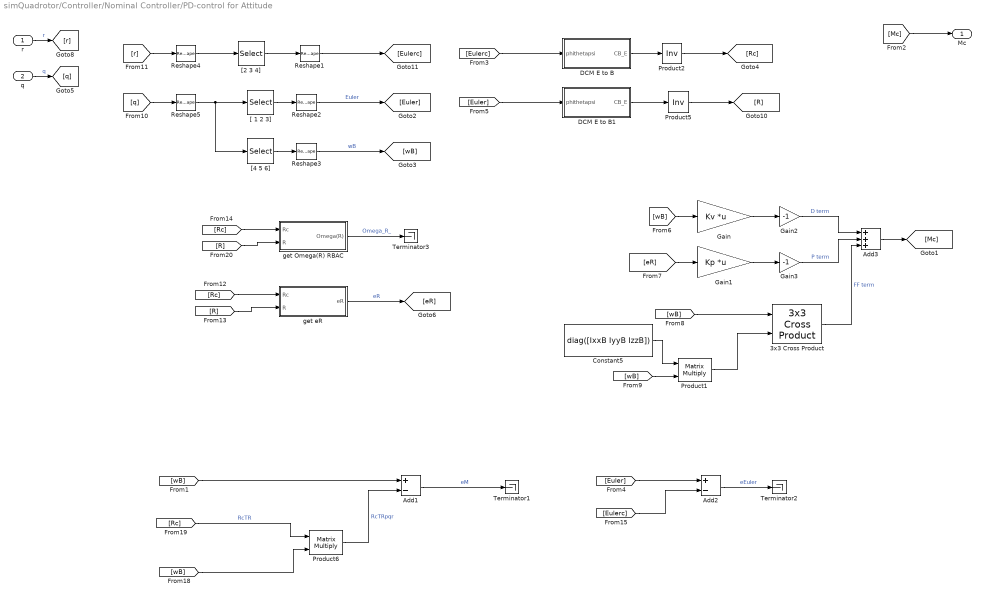
== system simQuadrotor/Controller/Nominal Controller/PD-control for Attitude ==
  r : Inport
  q : Inport  Port=2
  3x3 Cross Product : aerolibutil/3x3 Cross Product
  Add1 : Sum  Inputs=+-
  Add2 : Sum  Inputs=+-
  Add3 : Sum  Inputs=+++
  Constant5 : Constant  Value=diag([IxxB IyyB IzzB])  VectorParams1D=off
  DCM E to B : Subsystem
  DCM E to B1 : Subsystem
  Gain : Gain  Gain=Kv  Multiplication=Matrix(K*u)
  Gain1 : Gain  Gain=Kp  Multiplication=Matrix(K*u)
  Gain2 : Gain  Gain=-1
  Gain3 : Gain  Gain=-1
  Product1 : Product  Multiplication=Matrix(*)  RndMeth=Zero
  Product2 : Product  Inputs=/  Multiplication=Matrix(*)  RndMeth=Zero
  Product5 : Product  Inputs=/  Multiplication=Matrix(*)  RndMeth=Zero
  Product6 : Product  Multiplication=Matrix(*)  RndMeth=Zero
  Reshape{1..5} (5 alike) : Reshape  OutputDimensionality=Column vector (2-D)
  Terminator1 : Terminator
  Terminator2 : Terminator
  Terminator3 : Terminator
  "[ 1 2 3]" : Selector  NumberOfDimensions=2  InputPortWidth=3  IndexOptions=Index vector (dialog),Index vector (dialog)  Indices=[1 2 3],1  OutputSizes=1,1
  "[2 3 4]" : Selector  NumberOfDimensions=2  InputPortWidth=3  IndexOptions=Index vector (dialog),Index vector (dialog)  Indices=[2 3 4],1  OutputSizes=1,1
  "[4 5 6]" : Selector  NumberOfDimensions=2  InputPortWidth=3  IndexOptions=Index vector (dialog),Index vector (dialog)  Indices=[4 5 6],1  OutputSizes=1,1
  get Omega(R) RBAC : Subsystem
  get eR : Subsystem
  Mc : Outport
  wires:
  3x3 Cross Product/1 -> Add3/3  "FF term"
  Product1/1 -> 3x3 Cross Product/2
  [wB] -> Product1/2
  Constant5/1 -> Product1/1
  [wB] -> 3x3 Cross Product/1
  [R] -> get eR/2(R)
  get eR/1(eR) -> [eR]  "eR"
  [Rc] -> get eR/1(Rc)
  [R] -> get Omega(R) RBAC/2(R)
  Product5/1 -> [R]
  Product2/1 -> [Rc]
  [q] -> Reshape5/1
  "[ 1 2 3]"/1 -> Reshape2/1
  "[4 5 6]"/1 -> Reshape3/1
  Reshape5/1 -> "[ 1 2 3]"/1, "[4 5 6]"/1
  Add3/1 -> [Mc]
  Gain3/1 -> Add3/2  "P term"
  Gain2/1 -> Add3/1  "D term"
  [Rc] -> Product6/1  "RcTR"
  [wB] -> Product6/2
  [wB] -> Add1/1
  Product6/1 -> Add1/2  "RcTRpqr"
  Add1/1 -> Terminator1/1  "eM"
  [Euler] -> Add2/1
  [Eulerc] -> Add2/2
  Add2/1 -> Terminator2/1  "eEuler"
  [eR] -> Gain1/1
  [wB] -> Gain/1
  Gain/1 -> Gain2/1
  Gain1/1 -> Gain3/1
  get Omega(R) RBAC/1(Omega(R)) -> Terminator3/1  "Omega_R_"
  [Rc] -> get Omega(R) RBAC/1(Rc)
  Reshape1/1 -> [Eulerc]
  "[2 3 4]"/1 -> Reshape1/1
  [r] -> Reshape4/1
  Reshape2/1 -> [Euler]  "Euler"
  Reshape3/1 -> [wB]  "wB"
  Reshape4/1 -> "[2 3 4]"/1
  [Eulerc] -> DCM E to B/1(phithetapsi)
  DCM E to B/1(CB_E) -> Product2/1
  [Euler] -> DCM E to B1/1(phithetapsi)
  DCM E to B1/1(CB_E) -> Product5/1
  [Mc] -> Mc/1
  r/1 -> [r]  "r"
  q/1 -> [q]  "q"

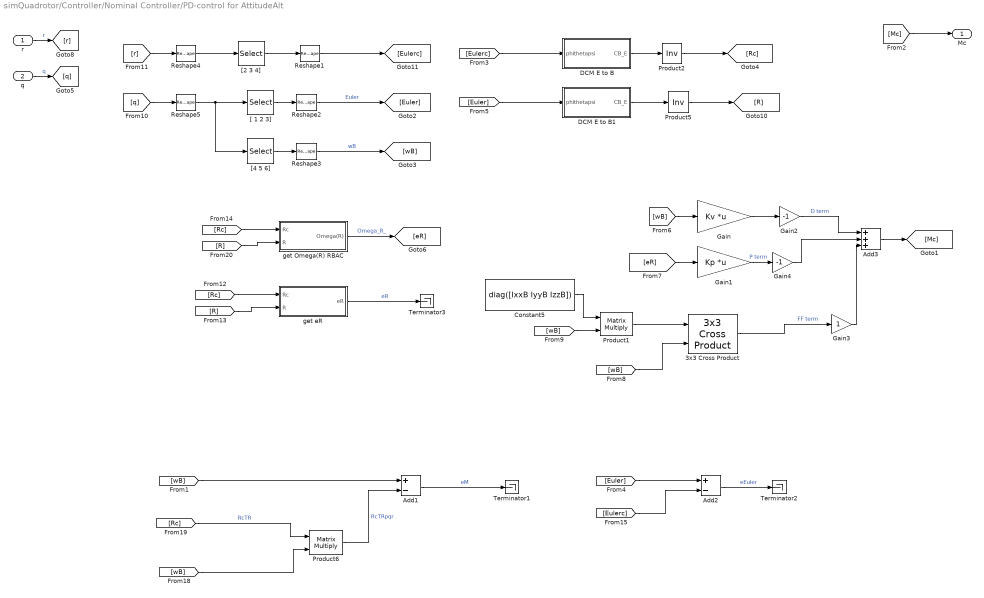
== system simQuadrotor/Controller/Nominal Controller/PD-control for AttitudeAlt ==
  r : Inport
  q : Inport  Port=2
  3x3 Cross Product : aerolibutil/3x3 Cross Product
  Add1 : Sum  Inputs=+-
  Add2 : Sum  Inputs=+-
  Add3 : Sum  Inputs=+++
  Constant5 : Constant  Value=diag([IxxB IyyB IzzB])  VectorParams1D=off
  DCM E to B : Subsystem
  DCM E to B1 : Subsystem
  Gain : Gain  Gain=Kv  Multiplication=Matrix(K*u)
  Gain1 : Gain  Gain=Kp  Multiplication=Matrix(K*u)
  Gain2 : Gain  Gain=-1
  Gain3 : Gain
  Gain4 : Gain  Gain=-1
  Product1 : Product  Multiplication=Matrix(*)  RndMeth=Zero
  Product2 : Product  Inputs=/  Multiplication=Matrix(*)  RndMeth=Zero
  Product5 : Product  Inputs=/  Multiplication=Matrix(*)  RndMeth=Zero
  Product6 : Product  Multiplication=Matrix(*)  RndMeth=Zero
  Reshape{1..5} (5 alike) : Reshape  OutputDimensionality=Column vector (2-D)
  Terminator1 : Terminator
  Terminator2 : Terminator
  Terminator3 : Terminator
  "[ 1 2 3]" : Selector  NumberOfDimensions=2  InputPortWidth=3  IndexOptions=Index vector (dialog),Index vector (dialog)  Indices=[1 2 3],1  OutputSizes=1,1
  "[2 3 4]" : Selector  NumberOfDimensions=2  InputPortWidth=3  IndexOptions=Index vector (dialog),Index vector (dialog)  Indices=[2 3 4],1  OutputSizes=1,1
  "[4 5 6]" : Selector  NumberOfDimensions=2  InputPortWidth=3  IndexOptions=Index vector (dialog),Index vector (dialog)  Indices=[4 5 6],1  OutputSizes=1,1
  get Omega(R) RBAC : Subsystem
  get eR : Subsystem
  Mc : Outport
  wires:
  q/1 -> [q]  "q"
  r/1 -> [r]  "r"
  [Mc] -> Mc/1
  DCM E to B1/1(CB_E) -> Product5/1
  [Euler] -> DCM E to B1/1(phithetapsi)
  DCM E to B/1(CB_E) -> Product2/1
  [Eulerc] -> DCM E to B/1(phithetapsi)
  Reshape4/1 -> "[2 3 4]"/1
  Reshape3/1 -> [wB]  "wB"
  Reshape2/1 -> [Euler]  "Euler"
  [r] -> Reshape4/1
  "[2 3 4]"/1 -> Reshape1/1
  Reshape1/1 -> [Eulerc]
  [Rc] -> get Omega(R) RBAC/1(Rc)
  Gain/1 -> Gain2/1
  [wB] -> Gain/1
  [eR] -> Gain1/1
  Add2/1 -> Terminator2/1  "eEuler"
  [Eulerc] -> Add2/2
  [Euler] -> Add2/1
  Add1/1 -> Terminator1/1  "eM"
  Product6/1 -> Add1/2  "RcTRpqr"
  [wB] -> Add1/1
  [wB] -> Product6/2
  [Rc] -> Product6/1  "RcTR"
  Gain2/1 -> Add3/1  "D term"
  Gain1/1 -> Gain4/1  "P term"
  Add3/1 -> [Mc]
  Reshape5/1 -> "[4 5 6]"/1, "[ 1 2 3]"/1
  "[4 5 6]"/1 -> Reshape3/1
  "[ 1 2 3]"/1 -> Reshape2/1
  [q] -> Reshape5/1
  Product2/1 -> [Rc]
  Product5/1 -> [R]
  [R] -> get Omega(R) RBAC/2(R)
  [Rc] -> get eR/1(Rc)
  [R] -> get eR/2(R)
  Constant5/1 -> Product1/1
  [wB] -> Product1/2
  3x3 Cross Product/1 -> Gain3/1  "FF term"
  get Omega(R) RBAC/1(Omega(R)) -> [eR]  "Omega_R_"
  get eR/1(eR) -> Terminator3/1  "eR"
  Gain3/1 -> Add3/3
  Gain4/1 -> Add3/2
  Product1/1 -> 3x3 Cross Product/1
  [wB] -> 3x3 Cross Product/2

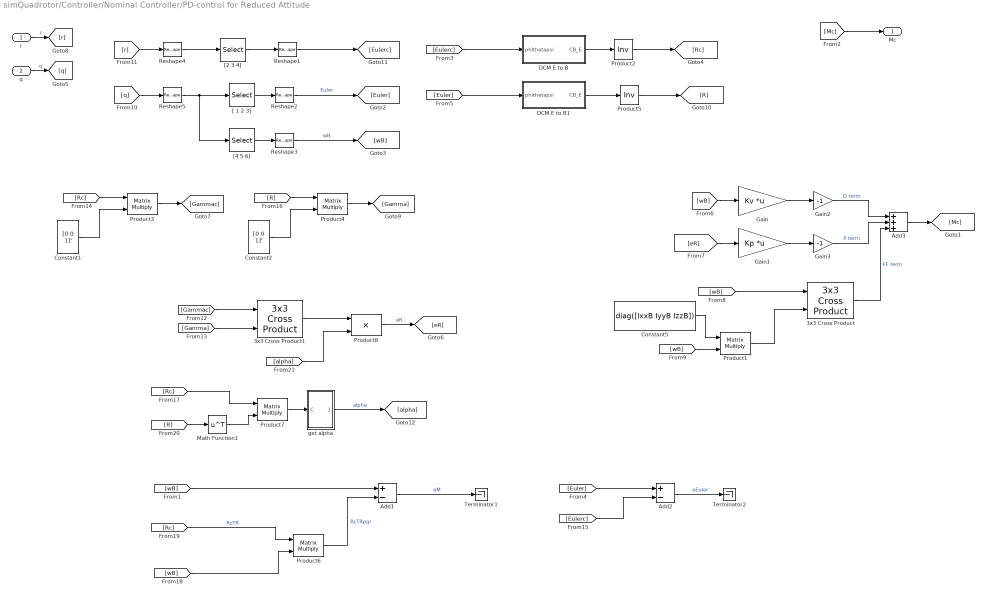
== system simQuadrotor/Controller/Nominal Controller/PD-control for Reduced Attitude ==
  r : Inport
  q : Inport  Port=2
  3x3 Cross Product : aerolibutil/3x3 Cross Product
  3x3 Cross Product1 : aerolibutil/3x3 Cross Product
  Add1 : Sum  Inputs=+-
  Add2 : Sum  Inputs=+-
  Add3 : Sum  Inputs=+++
  Constant1 : Constant  Value=[0 0 1]'  VectorParams1D=off
  Constant2 : Constant  Value=[0 0 1]'  VectorParams1D=off
  Constant5 : Constant  Value=diag([IxxB IyyB IzzB])  VectorParams1D=off
  DCM E to B : Subsystem
  DCM E to B1 : Subsystem
  Gain : Gain  Gain=Kv  Multiplication=Matrix(K*u)
  Gain1 : Gain  Gain=Kp  Multiplication=Matrix(K*u)
  Gain2 : Gain  Gain=-1
  Gain3 : Gain  Gain=-1
  Math Function1 : Math  Operator=transpose  SaturateOnIntegerOverflow=on
  Product{1,3..4,6..7} (5 alike) : Product  Multiplication=Matrix(*)  RndMeth=Zero
  Product2 : Product  Inputs=/  Multiplication=Matrix(*)  RndMeth=Zero
  Product5 : Product  Inputs=/  Multiplication=Matrix(*)  RndMeth=Zero
  Product8 : Product  RndMeth=Zero
  Reshape{1..5} (5 alike) : Reshape  OutputDimensionality=Column vector (2-D)
  Terminator1 : Terminator
  Terminator2 : Terminator
  "[ 1 2 3]" : Selector  NumberOfDimensions=2  InputPortWidth=3  IndexOptions=Index vector (dialog),Index vector (dialog)  Indices=[1 2 3],1  OutputSizes=1,1
  "[2 3 4]" : Selector  NumberOfDimensions=2  InputPortWidth=3  IndexOptions=Index vector (dialog),Index vector (dialog)  Indices=[2 3 4],1  OutputSizes=1,1
  "[4 5 6]" : Selector  NumberOfDimensions=2  InputPortWidth=3  IndexOptions=Index vector (dialog),Index vector (dialog)  Indices=[4 5 6],1  OutputSizes=1,1
  get alpha : Subsystem
  Mc : Outport
  wires:
  3x3 Cross Product/1 -> Add3/3  "FF term"
  Product1/1 -> 3x3 Cross Product/2
  [wB] -> Product1/2
  Constant5/1 -> Product1/1
  [wB] -> 3x3 Cross Product/1
  [Gamma] -> 3x3 Cross Product1/2
  [Gammac] -> 3x3 Cross Product1/1
  Product5/1 -> [R]
  Product2/1 -> [Rc]
  [q] -> Reshape5/1
  "[ 1 2 3]"/1 -> Reshape2/1
  "[4 5 6]"/1 -> Reshape3/1
  Reshape5/1 -> "[ 1 2 3]"/1, "[4 5 6]"/1
  Add3/1 -> [Mc]
  Gain3/1 -> Add3/2  "P term"
  Gain2/1 -> Add3/1  "D term"
  [Rc] -> Product6/1  "RcTR"
  [wB] -> Product6/2
  [wB] -> Add1/1
  Product6/1 -> Add1/2  "RcTRpqr"
  Add1/1 -> Terminator1/1  "eM"
  [Euler] -> Add2/1
  [Eulerc] -> Add2/2
  Add2/1 -> Terminator2/1  "eEuler"
  [eR] -> Gain1/1
  [wB] -> Gain/1
  Gain/1 -> Gain2/1
  Gain1/1 -> Gain3/1
  Reshape1/1 -> [Eulerc]
  "[2 3 4]"/1 -> Reshape1/1
  [r] -> Reshape4/1
  Reshape2/1 -> [Euler]  "Euler"
  Reshape3/1 -> [wB]  "wB"
  Reshape4/1 -> "[2 3 4]"/1
  [Eulerc] -> DCM E to B/1(phithetapsi)
  DCM E to B/1(CB_E) -> Product2/1
  [Euler] -> DCM E to B1/1(phithetapsi)
  DCM E to B1/1(CB_E) -> Product5/1
  [Mc] -> Mc/1
  r/1 -> [r]  "r"
  q/1 -> [q]  "q"
  [Rc] -> Product3/1
  Constant1/1 -> Product3/2
  Product3/1 -> [Gammac]
  [R] -> Product4/1
  Constant2/1 -> Product4/2
  Product4/1 -> [Gamma]
  get alpha/1(alpha) -> [alpha]  "alpha"
  [Rc] -> Product7/1
  [R] -> Math Function1/1
  Math Function1/1 -> Product7/2
  Product7/1 -> get alpha/1(C)
  3x3 Cross Product1/1 -> Product8/1
  Product8/1 -> [eR]  "eR"
  [alpha] -> Product8/2

== system simQuadrotor/Controller/Nominal Controller/PD-control for Reduced Attitude-Bullo ==
  r : Inport
  x : Inport  Port=2
  Add1 : Sum  Inputs=+-
  Constant1 : Constant  Value=0  VectorParams1D=off
  Gain4 : Gain  Gain=-1  Multiplication=Matrix(K*u)
  Gain5 : Gain  Gain=Kp4
  Gain6 : Gain  Gain=Kv4
  Math Function2 : Math  Operator=transpose  SaturateOnIntegerOverflow=on
  Math Function3 : Math  Operator=transpose  SaturateOnIntegerOverflow=on
  Mux : Mux  Inputs=2
  Mux1 : Mux  Inputs=2
  Mux2 : Mux  Inputs=2
  Product2 : Product  Multiplication=Matrix(*)  RndMeth=Zero
  Product3 : Product  Multiplication=Matrix(*)  RndMeth=Zero
  Product4 : Product  RndMeth=Zero
  Reshape{,1..4} (5 alike) : Reshape  OutputDimensionality=Column vector (2-D)
  "[4 5 6]" : Selector  InputPortWidth=6  Indices=4
  "[4 5 6]1" : Selector  InputPortWidth=6  Indices=5
  getRedAttRelatedPars : Subsystem
  Mc : Outport
  wires:
  r/1 -> [r]  "r"
  x/1 -> [x]  "x"
  [Mc] -> Mc/1  "Mc"
  [x] -> getRedAttRelatedPars/2(x)
  [r] -> getRedAttRelatedPars/1(r)
  getRedAttRelatedPars/2(dist_pi0_q) -> [dist_pi0_q]
  getRedAttRelatedPars/1(Yq_pi0) -> [Yq_pi0]
  getRedAttRelatedPars/3(pi1) -> [pi1]
  getRedAttRelatedPars/4(pi2) -> [pi2]
  [Yq_pi0] -> Math Function2/1
  Math Function2/1 -> Product2/1
  [pi2] -> Product2/2
  Product2/1 -> [V_Ypi2_V]
  [Yq_pi0] -> Math Function3/1
  Math Function3/1 -> Product3/1
  [pi1] -> Product3/2
  Product3/1 -> [V_Ypi1_V]
  Reshape3/1 -> [w1]  "w1"
  "[4 5 6]"/1 -> Reshape3/1
  [x] -> "[4 5 6]"/1
  Reshape1/1 -> [w2]  "w2"
  "[4 5 6]1"/1 -> Reshape1/1
  [x] -> "[4 5 6]1"/1
  [V_Ypi2_V] -> Gain4/1
  Gain4/1 -> Mux/1
  [V_Ypi1_V] -> Mux/2
  Mux/1 -> Reshape/1
  [dist_pi0_q] -> Product4/1
  Reshape/1 -> Product4/2
  Product4/1 -> Gain5/1
  Mux1/1 -> Reshape2/1
  [w1] -> Mux1/1
  [w2] -> Mux1/2
  Reshape2/1 -> Gain6/1
  Gain5/1 -> Add1/1  "Kpterm"
  Gain6/1 -> Add1/2  "Kvterm"
  Mux2/1 -> Reshape4/1
  Add1/1 -> Mux2/1
  Constant1/1 -> Mux2/2
  Reshape4/1 -> [Mc]

== system simQuadrotor/Controller/Nominal Controller/Propeller Rotation Rate Calculation ==
  fic : Inport
  Constant3 : Constant  Value=Kf
  Divide : Product  Inputs=*/
  Math Function : Math  Operator=sqrt  SaturateOnIntegerOverflow=on
  wc : Outport
  wires:
  Math Function/1 -> [wc]
  Divide/1 -> Math Function/1
  Constant3/1 -> Divide/2
  [fic] -> Divide/1
  [wc] -> wc/1
  fic/1 -> [fic]

== system simQuadrotor/Controller/Nominal Controller/Required Total Thrust ==
  q : Inport
  nc : Inport  Port=2
  Constant1 : Constant  Value=m
  Constant2 : Constant  Value=g
  Product of Elements : Product  Inputs=*
  Product1 : Product  RndMeth=Zero
  Product2 : Product  Inputs=**/  RndMeth=Zero
  Selector : Selector  NumberOfDimensions=2  InputPortWidth=3  IndexOptions=Index vector (dialog),Index vector (dialog)  Indices=[1 2],1  OutputSizes=1,1
  Trigonometric Function : Trigonometry  Operator=cos
  fc : Outport
  wires:
  [cosphi_costht] -> Product2/3
  Product1/1 -> Product2/2
  [nc] -> Product2/1
  nc/1 -> [nc]
  Trigonometric Function/1 -> Product of Elements/1
  Product of Elements/1 -> [cosphi_costht]
  Selector/1 -> Trigonometric Function/1
  Product2/1 -> fc/1
  Constant2/1 -> Product1/2
  Constant1/1 -> Product1/1
  q/1 -> Selector/1
